simulink model "rSpeedRegenDerate"  (R2024b)
settings: Solver=FixedStepAuto  StartTime=0.0  StopTime=10.0  RelTol=1e-3  EnableMultiTasking=on
libraries: simulink x1
settings Model: DataDictionary=Master_Dictionary.sldd  EnableAccessToBaseWorkspace=off  Creator=torni  LastModifiedBy=Will
settings OptimizationCC: DefaultParameterBehavior=Inlined  EnhancedBackFolding=on  PassReuseOutputArgsAs=Individual arguments  ZeroExternalMemoryAtStartup=off  ZeroInternalMemoryAtStartup=off  MaxStackSize=8192  OptimizeBlockOrder=speed  DifferentSizesBufferReuse=on  OptimizationCustomize=off  EfficientTunableParamExpr=on
settings DebuggingCC: ParameterTunabilityLossMsg=error
settings HardwareCC: ProdBitPerPointer=32  ProdBitPerSizeT=32  ProdBitPerPtrDiffT=32  ProdLargestAtomicInteger=Long  ProdLargestAtomicFloat=Double  ProdWordSize=32  ProdLongLongMode=on  ProdHWDeviceType=ARM Compatible->ARM Cortex-M
settings SFSimCC: MATLABDynamicMemAlloc=off
settings RTWCC: Description=Embedded Coder  SystemTargetFile=ert.tlc  HardwareBoard=STM32H7xx Based (Single-core)  TemplateMakefile=ert_default_tmf  Toolchain=GNU Tools for ARM Embedded Processors
settings CodeAppCC: ForceParamTrailComments=on  IgnoreCustomStorageClasses=off  OperatorAnnotations=on  SimulinkDataObjDesc=on  SFDataObjDesc=on  InsertBlockDesc=on
settings ERTTargetCC: TargetLangStandard=C99 (ISO)  CodeReplacementLibrary=ARM Cortex-M  ExtModeTransport=3  ExtModeStaticAlloc=on  ExtModeStaticAllocSize=2048  ExtModeMexFile=ext_xcp  ExtModeIntrfLevel=Level2 - Open

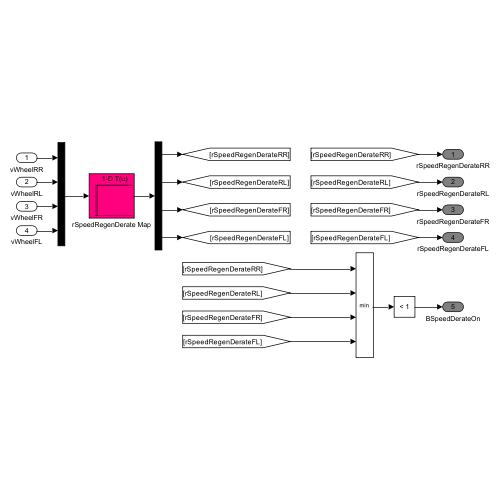
[thumbnail: Simulink's stored preview of the top-level diagram]
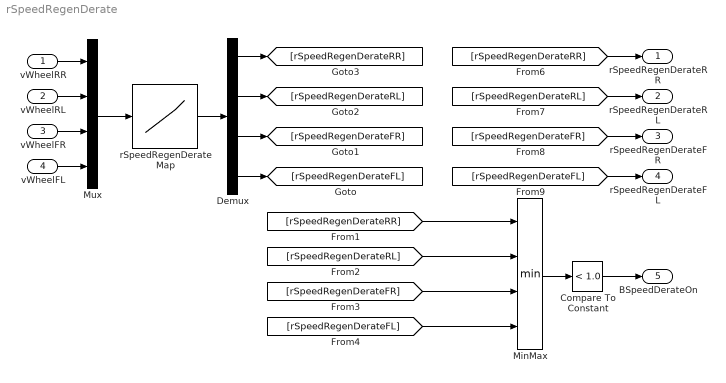
== system rSpeedRegenDerate ==
  vWheelRR : Inport  OutDataTypeStr=double
  vWheelRL : Inport  Port=2  OutDataTypeStr=double
  vWheelFR : Inport  Port=3  OutDataTypeStr=double
  vWheelFL : Inport  Port=4  OutDataTypeStr=double
  Compare To Constant : simulink/Logic and Bit Operations/Compare To Constant  relop=<  const=1.0  OutDataTypeStr=boolean
  Demux : Demux
  MinMax : MinMax  Inputs=4
  Mux : Mux
  rSpeedRegenDerate Map : Lookup_n-D  NumberOfTableDimensions=1  BreakpointsForDimension1=[0,3.9,4,100]  Table=[0,0,1,1]  InternalRulePriority=Speed  RndMeth=Simplest
  rSpeedRegenDerateRR : Outport  OutDataTypeStr=double  VectorParamsAs1DForOutWhenUnconnected=off
  rSpeedRegenDerateRL : Outport  Port=2  OutDataTypeStr=double  VectorParamsAs1DForOutWhenUnconnected=off
  rSpeedRegenDerateFR : Outport  Port=3  OutDataTypeStr=double  VectorParamsAs1DForOutWhenUnconnected=off
  rSpeedRegenDerateFL : Outport  Port=4  OutDataTypeStr=double  VectorParamsAs1DForOutWhenUnconnected=off
  BSpeedDerateOn : Outport  Port=5  OutDataTypeStr=boolean  VectorParamsAs1DForOutWhenUnconnected=off
  wires:
  [rSpeedRegenDerateRL] -> MinMax/2
  [rSpeedRegenDerateFL] -> MinMax/4
  Demux/3 -> [rSpeedRegenDerateFR]
  vWheelRL/1 -> Mux/2
  [rSpeedRegenDerateFR] -> MinMax/3
  Demux/4 -> [rSpeedRegenDerateFL]
  vWheelFL/1 -> Mux/4
  vWheelFR/1 -> Mux/3
  [rSpeedRegenDerateRR] -> MinMax/1
  Demux/1 -> [rSpeedRegenDerateRR]
  Compare To Constant/1 -> BSpeedDerateOn/1
  [rSpeedRegenDerateFL] -> rSpeedRegenDerateFL/1
  Demux/2 -> [rSpeedRegenDerateRL]
  vWheelRR/1 -> Mux/1
  [rSpeedRegenDerateRR] -> rSpeedRegenDerateRR/1
  rSpeedRegenDerate Map/1 -> Demux/1
  [rSpeedRegenDerateRL] -> rSpeedRegenDerateRL/1
  [rSpeedRegenDerateFR] -> rSpeedRegenDerateFR/1
  Mux/1 -> rSpeedRegenDerate Map/1
  MinMax/1 -> Compare To Constant/1
